simulink model "Ps1"  (R2020b)
settings: Solver=VariableStepAuto  StartTime=0.0  StopTime=10  RelTol=1e-3
libraries: simulink_extras x3
settings Model: Creator=prana  LastModifiedBy=prana

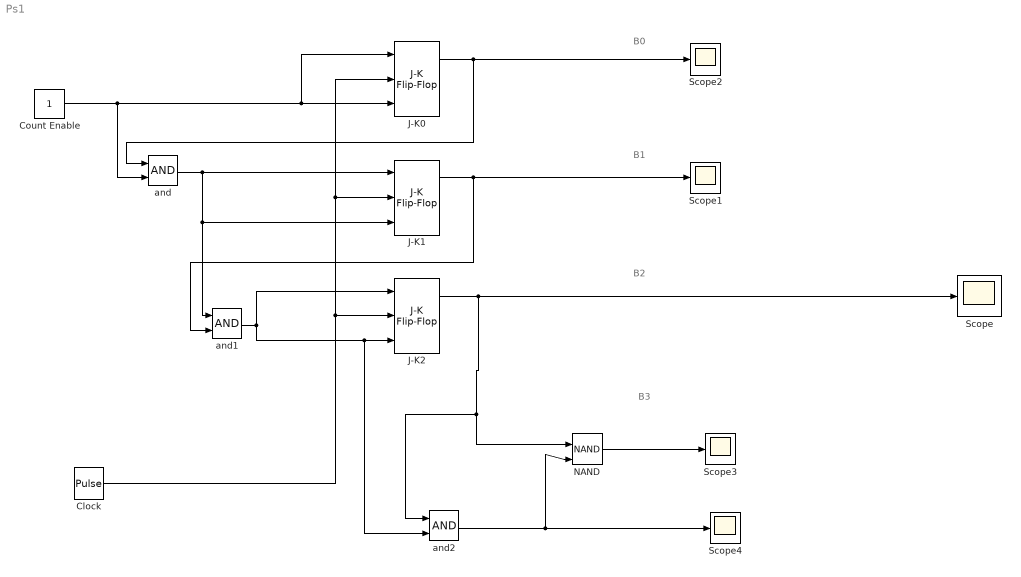
== system Ps1 ==
  note: B3
  note: B2
  note: B1
  note: B0
  Clock : DiscretePulseGenerator  PulseType=Time based  Period=1  PhaseDelay=1
  Count Enable : Constant  OutDataTypeStr=boolean
  J-K0 : simulink_extras/Flip Flops/J-K Flip-Flop  initial_condition=0
  J-K1 : simulink_extras/Flip Flops/J-K Flip-Flop  initial_condition=0
  J-K2 : simulink_extras/Flip Flops/J-K Flip-Flop  initial_condition=0
  NAND : Logic  Operator=NAND  IconShape=distinctive  AllPortsSameDT=off  OutDataTypeStr=boolean
  Scope{,1..4} (5 alike) : Scope
  and : Logic  AllPortsSameDT=off  OutDataTypeStr=boolean
  and1 : Logic  AllPortsSameDT=off  OutDataTypeStr=boolean
  and2 : Logic  AllPortsSameDT=off  OutDataTypeStr=boolean
  wires:
  J-K2/1 -> NAND/1, and2/1, Scope/1
  and1/1 -> J-K2/1, and2/2, J-K2/3
  and/1 -> J-K1/1, and1/1, J-K1/3
  J-K1/1 -> Scope1/1, and1/2
  Clock/1 -> J-K0/2, J-K1/2, J-K2/2
  J-K0/1 -> Scope2/1, and/1
  Count Enable/1 -> J-K0/3, J-K0/1, and/2
  and2/1 -> Scope4/1, NAND/2
  NAND/1 -> Scope3/1
